simulink model "Sigi_SIMO"  (R2019a)
settings: Solver=ode4  StartTime=0.0  StopTime=par.t_sim  FixedStep=par.Ts  MaxStep=1e-5  RelTol=1e-3
values from neighbouring files (symbols this model uses):
  d_p_0 = 0    [01_Sigi_v2_LQR_Design.m]
  d_theta_0 = 0    [01_Sigi_v2_LQR_Design.m]
  p_0 = 0    [01_Sigi_v2_LQR_Design.m]
  theta_0 = -25 /360*2*pi    (= -0.436332312999)    [01_Sigi_v2_LQR_Design.m]
undefined symbols (not defined in the file or in its folder): par
settings Model: Creator=Raffi  LastModifiedBy=Raffi
settings ModelReferenceCC: ModelReferenceMinAlgLoopOccurrences=on

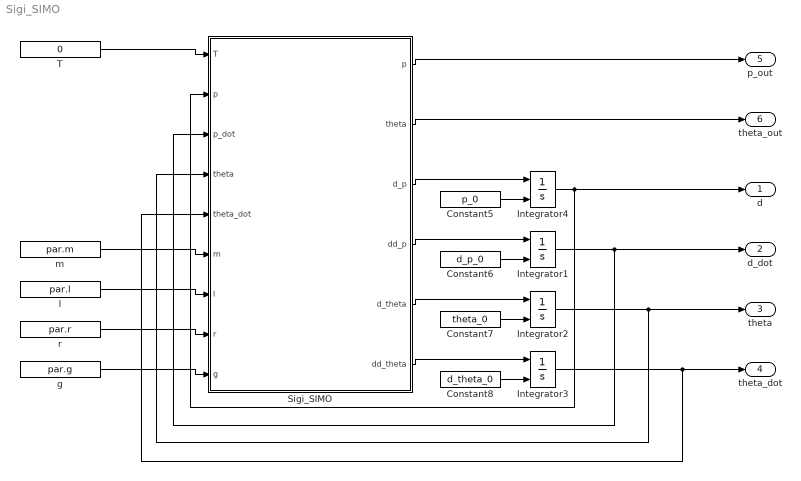
== system Sigi_SIMO ==
  Constant5 : Constant  Value=p_0
  Constant6 : Constant  Value=d_p_0
  Constant7 : Constant  Value=theta_0
  Constant8 : Constant  Value=d_theta_0
  Integrator{1..4} (4 alike) : Integrator  InitialConditionSource=external
  Sigi_SIMO : MATLAB Function  TreatAsAtomicUnit=on
  T : Constant  Value=0
  g : Constant  Value=par.g
  l : Constant  Value=par.l
  m : Constant  Value=par.m
  r : Constant  Value=par.r
  d : Outport
  d_dot : Outport  Port=2
  theta : Outport  Port=3
  theta_dot : Outport  Port=4
  p_out : Outport  Port=5
  theta_out : Outport  Port=6
  wires:
  Sigi_SIMO/5(d_theta) -> Integrator2/1
  Sigi_SIMO/6(dd_theta) -> Integrator3/1
  r/1 -> Sigi_SIMO/8(r)
  g/1 -> Sigi_SIMO/9(g)
  Sigi_SIMO/3(d_p) -> Integrator4/1
  Constant7/1 -> Integrator2/2
  Constant8/1 -> Integrator3/2
  Constant6/1 -> Integrator1/2
  m/1 -> Sigi_SIMO/6(m)
  Constant5/1 -> Integrator4/2
  Sigi_SIMO/4(dd_p) -> Integrator1/1
  Integrator4/1 -> Sigi_SIMO/2("p "), d/1
  Integrator3/1 -> theta_dot/1, Sigi_SIMO/5(theta_dot)
  Sigi_SIMO/1(p) -> p_out/1
  l/1 -> Sigi_SIMO/7(l)
  Sigi_SIMO/2(theta) -> theta_out/1
  Integrator1/1 -> d_dot/1, Sigi_SIMO/3(p_dot)
  Integrator2/1 -> Sigi_SIMO/4("theta "), theta/1
  T/1 -> Sigi_SIMO/1(T)

== matlab function Sigi_SIMO/Sigi_SIMO ==
  data: T input; p output; theta output; p input; d_p output; p_dot input; theta input; theta_dot input; dd_p output; d_theta output; dd_theta output; m input; l input; r input; g input
% This embedded Matlab function is only used to simulate an external Matlab
% function stored in a .m-file.
function    [p,theta,...                        % Sytem outputs
            d_p,dd_p,d_theta,dd_theta] = ...    % State updates
            Sigi_SIMO(...
            T,...                               % Sytem input
            p,p_dot,theta,theta_dot,...         % System states
            m, l, r, g)                         % System parameters


% Run external Matlab function
    [p,theta,...                        % Sytem outputs
    d_p,dd_p,d_theta,dd_theta] = ...    % State updates
    Sigi_SIMO_NonlinearODE(...
    T,...                               % Sytem input
    p,p_dot,theta,theta_dot,...         % System states
    m, l, r, g);                        % System parameters
